simulink model "kalman_filter"  (R2018a)
settings: Solver=FixedStepDiscrete  StartTime=0.0  StopTime=10.0  FixedStep=dt  RelTol=1e-3
model workspace (MAT data in the model file):
  P0 = Simulink.Parameter
  P0.Value = [1e-06  0  0; 0  1e-06  0; 0  0  1e-06]
  P0.DataType = 'auto'
  P0.Dimensions = [3 3]
  Q = Simulink.Parameter
  Q.Value = [3.49065850399e-09  0  0; 0  3.49065850399e-09  0; 0  0  3.49065850399e-09]
  Q.Description = 'Q = dt^4/4*acceleration covariance'
  Q.DataType = 'auto'
  Q.Dimensions = [3 3]
  R = Simulink.Parameter
  R.Value = [0.0174532925199  0  0; 0  0.0174532925199  0; 0  0  0.0174532925199]
  R.Description = 'sensor covariance'
  R.DataType = 'auto'
  R.Dimensions = [3 3]
  dt = Simulink.Parameter
  dt.Value = 0.02
  dt.DataType = 'double'
  dt.Dimensions = [1 1]
  nu = Simulink.Parameter
  nu.Value = [3 1]
  nu.DataType = 'auto'
  nu.Dimensions = [1 2]
  nz = Simulink.Parameter
  nz.Value = [3 1]
  nz.DataType = 'auto'
  nz.Dimensions = [1 2]
  x0 = Simulink.Parameter
  x0.Value = [0; 0; 0]
  x0.DataType = 'auto'
  x0.Dimensions = [3 1]
values from neighbouring files (symbols this model uses):
  dt = 1/100    (= 0.01)    [parameters.m]
  P0 = [1e-06 0 0;0 1e-06 0;0 0 1e-06]    [parameters.m]
  Q = diag([a*pqr_dot_covar(1)*a, a*pqr_dot_covar(2)*a, a*pqr_dot_covar(3)*a])    [parameters.m]
  R = diag([0.1, 0.1, 0.1])*9.81    [parameters.m]
  x0 = [0;0;0]    [parameters.m]
settings Model: ParameterArgumentNames=dt  OrderedModelArguments=off  Creator=Test  LastModifiedBy=Jason
settings DebuggingCC: AllowSymbolicDim=off

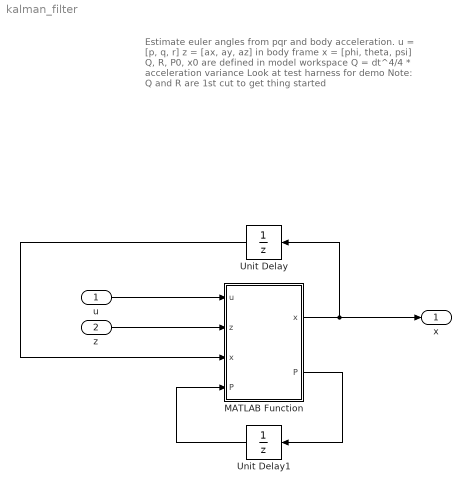
== system kalman_filter ==
  note: Estimate euler angles from pqr and body acceleration.
      |
      | u = [p, q, r]
      | z = [ax, ay, az] in body frame
      | x = [phi, theta, psi]
      |
      | Q, R, P0, x0 are defined in model workspace
      |
      | Q = dt^4/4 * acceleration variance
      |
      | Look at test harness for demo
      |
      | Note: Q and R are 1st cut to get thing started
  u : Inport  PortDimensions=nz
  z : Inport  Port=2  PortDimensions=nz
  MATLAB Function : MATLAB Function  TreatAsAtomicUnit=on  mask{Q=Q, R=R, dt=dt}
      mask prompts: dt "Sample Time"
  Unit Delay : UnitDelay  InitialCondition=x0  SampleTime=-1
  Unit Delay1 : UnitDelay  InitialCondition=P0  SampleTime=-1
  x : Outport
  wires:
  MATLAB Function/1(x) -> Unit Delay/1, x/1
  Unit Delay/1 -> MATLAB Function/3("x ")
  z/1 -> MATLAB Function/2(z)
  MATLAB Function/2(P) -> Unit Delay1/1
  Unit Delay1/1 -> MATLAB Function/4("P ")
  u/1 -> MATLAB Function/1(u)

== matlab function kalman_filter/MATLAB Function ==
  data: u input; z input; x input; x output; P output; P input; Q parameter; R parameter; dt parameter
function [x, P] = ekf(u, z, x, P, Q, R, dt)

[x, P] = predict(u, x, P, Q, dt);
[x, P] = update(z, x, P, R);

end

function [x, P] = predict(u, x, P, Q, dt)
% [x, P] = predict(u, x, P, Q, dt)
%
% predict states and covariance matrix using model

% nonlinear equation
x = eye(3,3)*x + euler2body(x)*dt*u;

F = Fj();
P = F*P*F'+Q;

end

function [x, P] = update(z, x, P, R)
% [x, P] = update(z, x, P, R)
%
% update states and covariance matrix using measurement

phi = x(1);
theta = x(2);
psi = x(3);

g = 9.81;
z_est = g*[
    -sin(theta);
    sin(phi)*cos(theta);
    cos(phi)*cos(theta)];
y = z - z_est;

H = Hj(x);
S = H*P*H'+R;
K = P*H'*inv(S);

nr = size(K,1);
nc = size(H,1);
x = x + K*y;
P = (eye(nr,nc)-K*H)*P;

end

function mat = Fj()
% Jacobian Matrix: F
%
% x' = Fx + Bu

mat = eye(3,3);

end

function mat = Bj(x, dt)
% Jacobian Matrix: B
%
% x' = Fx + Bu

dcm = euler2body(x);
mat = dt*dcm;

end

function mat = Hj(x)
% Jacobian Matrix: H
%
% z = Hx

phi = x(1);
theta = x(2);
psi = x(3);

g = 9.81;
mat = zeros(3,3);
mat(1,2) = -cos(theta);
mat(2,1) = cos(phi)*cos(theta);
mat(2,2) = -sin(phi)*sin(theta);
mat(3,1) = -sin(phi)*cos(theta);
mat(3,2) = -cos(phi)*sin(theta);
mat = g*mat;
end

function dcm = euler2body(euler)
phi = euler(1);
theta = euler(2);
psi = euler(3);

dcm = [
    1 sin(phi)*tan(theta) cos(phi)*tan(theta);
    0 cos(phi) -sin(phi);
    0 sin(phi)/cos(theta) cos(phi)/cos(theta)];
end
